simulink model "double_pendulum_model"  (R2022a)
settings: Solver=VariableStepAuto  StartTime=0.0  StopTime=10.0  MaxStep=1/60  RelTol=1e-3  AbsTol=1e-3  EnableMultiTasking=on
undefined symbols (not defined in the file): X, Y, Z
libraries: sm_lib x15, nesl_utility x9, slpidlib x2
settings Model: Creator=tripa  LastModifiedBy=tripa
settings SolverCC: AutoScaleAbsTol=off  AlgebraicLoopSolver=TrustRegion  MaxZcPerStep=1
settings DataIOCC: LimitDataPoints=on  MaxDataPoints=10000
settings OptimizationCC: LifeSpan=inf
settings DebuggingCC: UnconnectedInputMsg=warning  UnconnectedOutputMsg=warning  UnconnectedLineMsg=warning  AllowSymbolicDim=off  SFUnexpectedBacktrackingDiag=warning  SFNoUnconditionalDefaultTransitionDiag=warning  SFExecutionAtInitializationDiag=none  SFMachineParentedDataDiag=warning  ArithmeticOperatorsInVariantConditions=warning
settings SFSimCC: SimUseLocalCustomCode=off  CustomCodeUndefinedFunction=UseInterfaceOnly
settings RTWCC: RTWUseLocalCustomCode=off  DLArmComputeVersion=19.05
settings CodeAppCC: StateflowObjectComments=on
settings GRTTargetCC: TargetLangStandard=C89/C90 (ANSI)
settings ConfigComp: CovMetricSettings=dw  CovSaveCumulativeToWorkspaceVar=on  CovSaveSingleToWorkspaceVar=on  CovExternalEMLEnable=off  CovSFcnEnable=off
settings SimscapeCC: SimscapeLogType=all  SimscapeLogSimulationStatistics=on  SimscapeLogDataHistory=10000

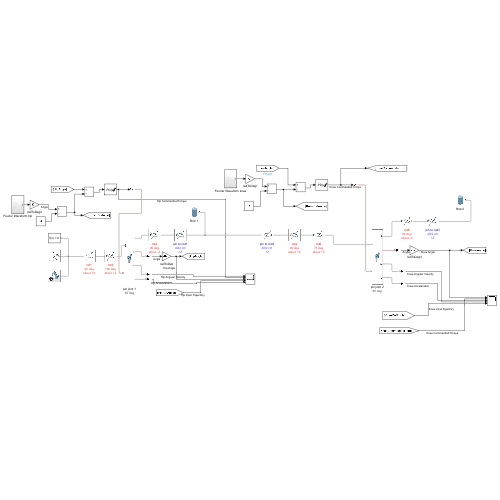
[thumbnail: Simulink's stored preview of the top-level diagram]
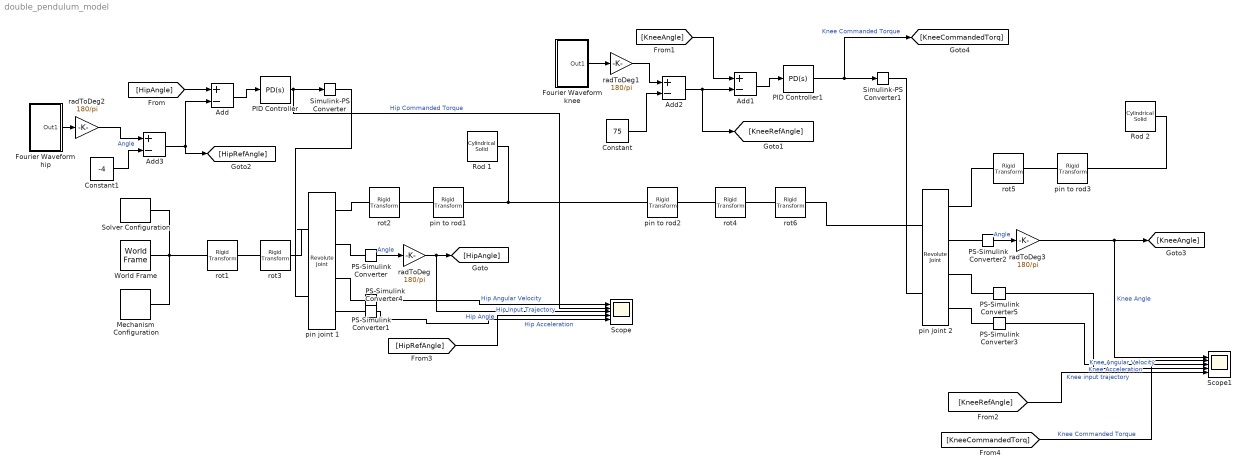
== system double_pendulum_model ==
  Add{,1..3} (4 alike) : Sum  Inputs=+-
  Constant : Constant  Value=75  SampleTime=-1
  Constant1 : Constant  Value=-4  SampleTime=-1
  Fourier Waveform hip : Subsystem
  Fourier Waveform knee : Subsystem
  Mechanism Configuration : sm_lib/Utilities/Mechanism Configuration  UniformGravity=Constant  GravityVector=[0 0 -9.81]  GravityUnits=m/s^2  LinearizationDelta=0.001  JointModeTransitionNonlinearIterations=2
  PID Controller : slpidlib/PID Controller  Controller=PD  Form=Parallel  TimeDomain=Continuous-time  UseExternalTs=off  SampleTime=-1  IntegratorMethod=Forward Euler  FilterMethod=Forward Euler  ControllerParametersSource=internal  P=-23.3308490537665  I=-3.87247530193336  UseKiTs=off  D=-1.5  N=1747.15655402676  UseFilter=on  TunerSelectOption=Transfer Function Based (PID Tuner App)  InitialConditionSource=internal  InitialConditionForIntegrator=0  InitialConditionForFilter=0  DifferentiatorICPrevScaledInput=0  ExternalReset=none  TrackingMode=off  Kt=1  LimitOutput=on  SatLimitsSource=internal  UpperSaturationLimit=20  LowerSaturationLimit=-20  LinearizeAsGain=on  AntiWindupMode=none  Kb=1  POutMin=[]  POutMax=[]  IOutMin=[]  IOutMax=[]  DOutMin=[]  DOutMax=[]  NOutMin=[]  NOutMax=[]  SumOutMin=[]  SumOutMax=[]  SaturationOutMin=[]  SaturationOutMax=[]  PParamMin=[]  PParamMax=[]  IParamMin=[]  IParamMax=[]  DParamMin=[]  DParamMax=[]  NParamMin=[]  NParamMax=[]  KbParamMin=[]  KbParamMax=[]  KtParamMin=[]  KtParamMax=[]  KbOutMin=[]  KbOutMax=[]  KtOutMin=[]  KtOutMax=[]  IntegratorOutMin=[]  IntegratorOutMax=[]  FilterOutMin=[]  FilterOutMax=[]  SumI1OutMin=[]  SumI1OutMax=[]  SumI2OutMin=[]  SumI2OutMax=[]  SumI3OutMin=[]  SumI3OutMax=[]  SumI4OutMin=[]  SumI4OutMax=[]  SumDOutMin=[]  SumDOutMax=[]  DifferentiatorOutMin=[]  DifferentiatorOutMax=[]  FilterDiffOutCoefMin=[]  FilterDiffOutCoefMax=[]  ReciprocalOutMin=[]  ReciprocalOutMax=[]  SumDenOutMin=[]  SumDenOutMax=[]  SumNumOutMin=[]  SumNumOutMax=[]  DivideOutMin=[]  DivideOutMax=[]  UdiffTsProdOutMin=[]  UdiffTsProdOutMax=[]  NTsProdOutMin=[]  NTsProdOutMax=[]  UintegralTsProdOutMin=[]  UintegralTsProdOutMax=[]  UngainTsProdOutMin=[]  UngainTsProdOutMax=[]  IntegratorContinuousStateAttributes=''  IntegratorStateMustResolveToSignalObject=off  IntegratorRTWStateStorageClass=Auto  FilterContinuousStateAttributes=''  FilterStateMustResolveToSignalObject=off  FilterRTWStateStorageClass=Auto  ParallelPVariant=InternalParameters  IdealPVariant=Disabled  IVariant=Disabled  DVariant=InternalParameters  IntegratorVariant=Disabled  SatVariant=Enabled  AWVariant=Disabled  PCopyVariant=Disabled  TRVariant=Disabled  FdbkBlocksVariant=Forward  IdealPFdbkVariant=Disabled  SatFdbkVariant=Disabled  DerivativeFilterVariant=ContFilter  NVariant=InternalParameters  NCopyVariant=Disabled  FilterICVariant=InternalICsFilter  IntegratorICVariant=Disabled  ExternalResetVariant=Disabled  TRSumVariant=Passthrough  SumFdbkVariant=Disabled  SumVariant=Sum_PD  TsampFilterVariant=InternalTs  TsampNgainVariant=Passthrough  TsampIntegralVariant=Disabled_SignalSpec  ExternalSaturationOutDataTypeStr=Inherit: Same as second input  aMode=0
  PID Controller1 : slpidlib/PID Controller  Controller=PD  Form=Parallel  TimeDomain=Continuous-time  UseExternalTs=off  SampleTime=-1  IntegratorMethod=Forward Euler  FilterMethod=Forward Euler  ControllerParametersSource=internal  P=-24.553266008043  I=-3.87247530193336  UseKiTs=off  D=-0.217820826801744  N=2156.83917251684  UseFilter=on  TunerSelectOption=Transfer Function Based (PID Tuner App)  InitialConditionSource=internal  InitialConditionForIntegrator=0  InitialConditionForFilter=0  DifferentiatorICPrevScaledInput=0  ExternalReset=none  TrackingMode=off  Kt=1  LimitOutput=on  SatLimitsSource=internal  UpperSaturationLimit=15  LowerSaturationLimit=-15  LinearizeAsGain=on  AntiWindupMode=none  Kb=1  POutMin=[]  POutMax=[]  IOutMin=[]  IOutMax=[]  DOutMin=[]  DOutMax=[]  NOutMin=[]  NOutMax=[]  SumOutMin=[]  SumOutMax=[]  SaturationOutMin=[]  SaturationOutMax=[]  PParamMin=[]  PParamMax=[]  IParamMin=[]  IParamMax=[]  DParamMin=[]  DParamMax=[]  NParamMin=[]  NParamMax=[]  KbParamMin=[]  KbParamMax=[]  KtParamMin=[]  KtParamMax=[]  KbOutMin=[]  KbOutMax=[]  KtOutMin=[]  KtOutMax=[]  IntegratorOutMin=[]  IntegratorOutMax=[]  FilterOutMin=[]  FilterOutMax=[]  SumI1OutMin=[]  SumI1OutMax=[]  SumI2OutMin=[]  SumI2OutMax=[]  SumI3OutMin=[]  SumI3OutMax=[]  SumI4OutMin=[]  SumI4OutMax=[]  SumDOutMin=[]  SumDOutMax=[]  DifferentiatorOutMin=[]  DifferentiatorOutMax=[]  FilterDiffOutCoefMin=[]  FilterDiffOutCoefMax=[]  ReciprocalOutMin=[]  ReciprocalOutMax=[]  SumDenOutMin=[]  SumDenOutMax=[]  SumNumOutMin=[]  SumNumOutMax=[]  DivideOutMin=[]  DivideOutMax=[]  UdiffTsProdOutMin=[]  UdiffTsProdOutMax=[]  NTsProdOutMin=[]  NTsProdOutMax=[]  UintegralTsProdOutMin=[]  UintegralTsProdOutMax=[]  UngainTsProdOutMin=[]  UngainTsProdOutMax=[]  IntegratorContinuousStateAttributes=''  IntegratorStateMustResolveToSignalObject=off  IntegratorRTWStateStorageClass=Auto  FilterContinuousStateAttributes=''  FilterStateMustResolveToSignalObject=off  FilterRTWStateStorageClass=Auto  ParallelPVariant=InternalParameters  IdealPVariant=Disabled  IVariant=Disabled  DVariant=InternalParameters  IntegratorVariant=Disabled  SatVariant=Enabled  AWVariant=Disabled  PCopyVariant=Disabled  TRVariant=Disabled  FdbkBlocksVariant=Forward  IdealPFdbkVariant=Disabled  SatFdbkVariant=Disabled  DerivativeFilterVariant=ContFilter  NVariant=InternalParameters  NCopyVariant=Disabled  FilterICVariant=InternalICsFilter  IntegratorICVariant=Disabled  ExternalResetVariant=Disabled  TRSumVariant=Passthrough  SumFdbkVariant=Disabled  SumVariant=Sum_PD  TsampFilterVariant=InternalTs  TsampNgainVariant=Passthrough  TsampIntegralVariant=Disabled_SignalSpec  ExternalSaturationOutDataTypeStr=Inherit: Same as second input  aMode=0
  PS-Simulink Converter{,1..5} (6 alike) : nesl_utility/PS-Simulink Converter  PhysicalDomain=network_engine_domain  SubClassName=ps_output  LeftPortType=input  RightPortType=output  PseudoPeriodic=off  Frequencies=[]  VectorFormat=inherit  Unit=inherit  AffineConversion=off
      settings: SourceProductBaseCode=SS,PW,VE
  Rod 1 : sm_lib/Body Elements/Cylindrical Solid  GraphicAmbientColor=[0.15 0.15 0.15 1.0]  BasedOnType=Density  CenterOfMass=[0 0 0]  CenterOfMassUnits=m  GraphicDiffuseColor=[0.5 0.5 0.5]  CylinderLength=40  CylinderLengthUnits=cm  CylinderRadius=3  CylinderRadiusUnits=cm  Density=2700  DensityUnits=kg/m^3  DoExposeReferenceFrame=on  GraphicEmissiveColor=[0.0 0.0 0.0 1.0]  ExportEntireGeometry=off  SerializedFrames=<Frames/>  MarkerShape=Sphere  MarkerSize=10  GraphicType=FromGeometry  InertiaType=CalculateFromGeometry  Mass=1  MassUnits=kg  MomentsOfInertia=[1 1 1]  MomentsOfInertiaUnits=kg*m^2  GraphicOpacity=1.0  ProductsOfInertia=[0 0 0]  ProductsOfInertiaUnits=kg*m^2  GraphicShininess=75  GraphicSpecularColor=[0.5 0.5 0.5 1.0]  GraphicVisPropType=SimpleVisualProperties
  Rod 2 : sm_lib/Body Elements/Cylindrical Solid  GraphicAmbientColor=[0.15 0.15 0.15 1.0]  BasedOnType=Density  CenterOfMass=[0 0 0]  CenterOfMassUnits=m  GraphicDiffuseColor=[0.5 0.5 0.5]  CylinderLength=40  CylinderLengthUnits=cm  CylinderRadius=3  CylinderRadiusUnits=cm  Density=2700  DensityUnits=kg/m^3  DoExposeReferenceFrame=on  GraphicEmissiveColor=[0.0 0.0 0.0 1.0]  ExportEntireGeometry=off  SerializedFrames=<Frames/>  MarkerShape=Sphere  MarkerSize=10  GraphicType=FromGeometry  InertiaType=CalculateFromGeometry  Mass=1  MassUnits=kg  MomentsOfInertia=[1 1 1]  MomentsOfInertiaUnits=kg*m^2  GraphicOpacity=1.0  ProductsOfInertia=[0 0 0]  ProductsOfInertiaUnits=kg*m^2  GraphicShininess=75  GraphicSpecularColor=[0.5 0.5 0.5 1.0]  GraphicVisPropType=SimpleVisualProperties
  Scope : Scope  NumInputPorts=5
  Scope1 : Scope  NumInputPorts=5
  Simulink-PS Converter : nesl_utility/Simulink-PS Converter  PhysicalDomain=network_engine_domain  SubClassName=ps_input  LeftPortType=input  RightPortType=output  PseudoPeriodic=off  Frequencies=[]  NoiseDistribution=none  NoiseParameters=[]  Unit=1  AffineConversion=off  FilteringAndDerivatives=provide  SimscapeFilterOrder=1  InputFilterTimeConstant=0.001  UdotUserProvided=0
      settings: SourceProductBaseCode=SS,PW,VE
  Simulink-PS Converter1 : nesl_utility/Simulink-PS Converter  PhysicalDomain=network_engine_domain  SubClassName=ps_input  LeftPortType=input  RightPortType=output  PseudoPeriodic=off  Frequencies=[]  NoiseDistribution=none  NoiseParameters=[]  Unit=1  AffineConversion=off  FilteringAndDerivatives=provide  SimscapeFilterOrder=1  InputFilterTimeConstant=0.001  UdotUserProvided=0
      settings: SourceProductBaseCode=SS,PW,VE
  Solver Configuration : nesl_utility/Solver Configuration  PhysicalDomain=network_engine_domain  SubClassName=solver  LeftPortType=input  RightPortType=generic  Tones=[]  Harmonics=[]  SimulateNoise=off  Profile=off  UseLocalSampling=off  EnableSwitchedLinearOptims=on  FrequencyDomain=off  UseCCode=off  RelTol=0.001  AbsTol=1e-06  MinStep=1e-09  ToWorkspace=off  RevertToSquareIcSolve=off  NumHomotopyIterations=100  PhasorMode=off  PhasorModeNumHarmonics=1  IndexReductionMethod=DerivativeReplacement  DoDC=off  ResidualTolerance=1e-09  UseLocalSolver=off  LocalSolverChoice=NE_BACKWARD_EULER_ADVANCER  LocalSolverSampleTime=0.001  DoFixedCost=off  MaxNonlinIter=3  MaxModeIter=2  ComputeImpulses=off  ImpulseIterations=2  LinearAlgebra=Sparse  LinearAlgebraNumThread=0  EquationFormulation=NE_TIME_EF  DelaysMemoryBudget=1024  AutomaticFiltering=on  FilteringTimeConstant=0.001  PartitionStorageMethod=AS_NEEDED  PartitionMemoryBudget=1024  PartitionMethod=FAST
      settings: SourceProductBaseCode=SS,PW,VE
  World Frame : sm_lib/Frames and Transforms/World Frame
  pin joint 1 : sm_lib/Joints/Revolute Joint  JointMode=Normal  SenseConstraintForce=off  SenseConstraintForceX=off  SenseConstraintForceY=off  SenseConstraintForceZ=off  SenseConstraintTorque=off  SenseConstraintTorqueX=off  SenseConstraintTorqueY=off  SenseConstraintTorqueZ=off  SenseTotalForce=off  SenseTotalForceX=off  SenseTotalForceY=off  SenseTotalForceZ=off  SenseTotalTorque=off  SenseTotalTorqueX=off  SenseTotalTorqueY=off  SenseTotalTorqueZ=off  CompositeWrenchDir=FollowerOnBase  CompositeWrenchFrame=BaseFrame  EquilibriumPosition=0  EquilibriumPositionUnits=deg  SpringStiffness=0  SpringStiffnessUnits=N*m/deg  DampingCoefficient=0  DampingCoefficientUnits=N*m/(deg/s)  TorqueActuationMode=InputTorque  MotionActuationMode=ComputedMotion  SensePosition=on  SenseVelocity=on  SenseAcceleration=on  SenseTorqueForce=off  SenseLowerLimitTorqueForce=off  SenseUpperLimitTorqueForce=off  LowerLimitSpecify=off  LowerLimitBound=-90  LowerLimitBoundUnits=deg  LowerLimitStiffness=1e4  LowerLimitStiffnessUnits=N*m/deg  LowerLimitDamping=10  LowerLimitDampingUnits=N*m/(deg/s)  LowerLimitTransitionRegionWidth=0.1  LowerLimitTransitionRegionWidthUnits=deg  UpperLimitSpecify=off  UpperLimitBound=90  UpperLimitBoundUnits=deg  UpperLimitStiffness=1e4  UpperLimitStiffnessUnits=N*m/deg  UpperLimitDamping=10  UpperLimitDampingUnits=N*m/(deg/s)  UpperLimitTransitionRegionWidth=0.1  UpperLimitTransitionRegionWidthUnits=deg  PositionTargetSpecify=off  PositionTargetPriority=High  PositionTargetValue=90  PositionTargetValueUnits=deg  VelocityTargetSpecify=off  VelocityTargetPriority=High  VelocityTargetValue=0  VelocityTargetValueUnits=deg/s
      settings: AttributesFormatString=%<PositionTargetValue> %<PositionTargetValueUnits>
  pin joint 2 : sm_lib/Joints/Revolute Joint  JointMode=Normal  SenseConstraintForce=off  SenseConstraintForceX=off  SenseConstraintForceY=off  SenseConstraintForceZ=off  SenseConstraintTorque=off  SenseConstraintTorqueX=off  SenseConstraintTorqueY=off  SenseConstraintTorqueZ=off  SenseTotalForce=off  SenseTotalForceX=off  SenseTotalForceY=off  SenseTotalForceZ=off  SenseTotalTorque=off  SenseTotalTorqueX=off  SenseTotalTorqueY=off  SenseTotalTorqueZ=off  CompositeWrenchDir=FollowerOnBase  CompositeWrenchFrame=BaseFrame  EquilibriumPosition=0  EquilibriumPositionUnits=deg  SpringStiffness=0  SpringStiffnessUnits=N*m/deg  DampingCoefficient=0  DampingCoefficientUnits=N*m/(deg/s)  TorqueActuationMode=InputTorque  MotionActuationMode=ComputedMotion  SensePosition=on  SenseVelocity=on  SenseAcceleration=on  SenseTorqueForce=off  SenseLowerLimitTorqueForce=off  SenseUpperLimitTorqueForce=off  LowerLimitSpecify=off  LowerLimitBound=-90  LowerLimitBoundUnits=deg  LowerLimitStiffness=1e4  LowerLimitStiffnessUnits=N*m/deg  LowerLimitDamping=10  LowerLimitDampingUnits=N*m/(deg/s)  LowerLimitTransitionRegionWidth=0.1  LowerLimitTransitionRegionWidthUnits=deg  UpperLimitSpecify=off  UpperLimitBound=90  UpperLimitBoundUnits=deg  UpperLimitStiffness=1e4  UpperLimitStiffnessUnits=N*m/deg  UpperLimitDamping=10  UpperLimitDampingUnits=N*m/(deg/s)  UpperLimitTransitionRegionWidth=0.1  UpperLimitTransitionRegionWidthUnits=deg  PositionTargetSpecify=off  PositionTargetPriority=High  PositionTargetValue=90  PositionTargetValueUnits=deg  VelocityTargetSpecify=off  VelocityTargetPriority=High  VelocityTargetValue=0  VelocityTargetValueUnits=deg/s
      settings: AttributesFormatString=%<PositionTargetValue> %<PositionTargetValueUnits>
  pin to rod1 : sm_lib/Frames and Transforms/Rigid Transform  TranslationMethod=StandardAxis  TranslationStandardOffset=40/2  TranslationLengthUnit=cm  TranslationStandardAxis=+Z  TranslationCartesianOffset=[0 0 0]  TranslationROffset=0  TranslationROffsetUnits=m  TranslationZOffset=0  TranslationZOffsetUnits=m  TranslationThetaOffset=0  TranslationThetaOffsetUnits=deg  RotationMethod=None  RotationAngleUnits=deg  RotationStandardAxis=+X  RotationAngle=90  RotationArbitraryAxis=[0 0 1]  FollAlignAxisA=+X  BaseAlignAxisA=+Y  FollAlignAxisB=+Y  BaseAlignAxisB=+Z  RotationSequenceAxes=FollowerAxes  RotationSequence=XYX  RotationSequenceAngles=[0 0 0]  RotationSequenceAnglesUnits=deg  RotationMatrix=[1 0 0; 0 1 0; 0 0 1]
      settings: AttributesFormatString=|
      | %<TranslationStandardOffset> %<TranslationLengthUnit>
      | %<TranslationStandardAxis>
  pin to rod2 : sm_lib/Frames and Transforms/Rigid Transform  TranslationMethod=StandardAxis  TranslationStandardOffset=40/2  TranslationLengthUnit=cm  TranslationStandardAxis=+Z  TranslationCartesianOffset=[0 0 0]  TranslationROffset=0  TranslationROffsetUnits=m  TranslationZOffset=0  TranslationZOffsetUnits=m  TranslationThetaOffset=0  TranslationThetaOffsetUnits=deg  RotationMethod=None  RotationAngleUnits=deg  RotationStandardAxis=+X  RotationAngle=90  RotationArbitraryAxis=[0 0 1]  FollAlignAxisA=+X  BaseAlignAxisA=+Y  FollAlignAxisB=+Y  BaseAlignAxisB=+Z  RotationSequenceAxes=FollowerAxes  RotationSequence=XYX  RotationSequenceAngles=[0 0 0]  RotationSequenceAnglesUnits=deg  RotationMatrix=[1 0 0; 0 1 0; 0 0 1]
      settings: AttributesFormatString=|
      | %<TranslationStandardOffset> %<TranslationLengthUnit>
      | %<TranslationStandardAxis>
  pin to rod3 : sm_lib/Frames and Transforms/Rigid Transform  TranslationMethod=StandardAxis  TranslationStandardOffset=40/2  TranslationLengthUnit=cm  TranslationStandardAxis=+Z  TranslationCartesianOffset=[0 0 0]  TranslationROffset=0  TranslationROffsetUnits=m  TranslationZOffset=0  TranslationZOffsetUnits=m  TranslationThetaOffset=0  TranslationThetaOffsetUnits=deg  RotationMethod=None  RotationAngleUnits=deg  RotationStandardAxis=+X  RotationAngle=90  RotationArbitraryAxis=[0 0 1]  FollAlignAxisA=+X  BaseAlignAxisA=+Y  FollAlignAxisB=+Y  BaseAlignAxisB=+Z  RotationSequenceAxes=FollowerAxes  RotationSequence=XYX  RotationSequenceAngles=[0 0 0]  RotationSequenceAnglesUnits=deg  RotationMatrix=[1 0 0; 0 1 0; 0 0 1]
      settings: AttributesFormatString=|
      | %<TranslationStandardOffset> %<TranslationLengthUnit>
      | %<TranslationStandardAxis>
  radToDeg{,1..3} (4 alike) : Gain  Gain=180/pi
  rot1 : sm_lib/Frames and Transforms/Rigid Transform  TranslationMethod=None  TranslationStandardOffset=0  TranslationLengthUnit=m  TranslationStandardAxis=+Z  TranslationCartesianOffset=[0 0 0]  TranslationROffset=0  TranslationROffsetUnits=m  TranslationZOffset=0  TranslationZOffsetUnits=m  TranslationThetaOffset=0  TranslationThetaOffsetUnits=deg  RotationMethod=StandardAxis  RotationAngleUnits=deg  RotationStandardAxis=+X  RotationAngle=90  RotationArbitraryAxis=[0 0 1]  FollAlignAxisA=+X  BaseAlignAxisA=+Y  FollAlignAxisB=+Y  BaseAlignAxisB=+Z  RotationSequenceAxes=FollowerAxes  RotationSequence=XYX  RotationSequenceAngles=[0 0 0]  RotationSequenceAnglesUnits=deg  RotationMatrix=[1 0 0; 0 1 0; 0 0 1]
      settings: AttributesFormatString=|
      | %<RotationAngle> %<RotationAngleUnits>
      | about %<RotationStandardAxis>
  rot2 : sm_lib/Frames and Transforms/Rigid Transform  TranslationMethod=None  TranslationStandardOffset=0  TranslationLengthUnit=m  TranslationStandardAxis=+Z  TranslationCartesianOffset=[0 0 0]  TranslationROffset=0  TranslationROffsetUnits=m  TranslationZOffset=0  TranslationZOffsetUnits=m  TranslationThetaOffset=0  TranslationThetaOffsetUnits=deg  RotationMethod=StandardAxis  RotationAngleUnits=deg  RotationStandardAxis=-X  RotationAngle=90  RotationArbitraryAxis=[0 0 1]  FollAlignAxisA=+X  BaseAlignAxisA=+Y  FollAlignAxisB=+Y  BaseAlignAxisB=+Z  RotationSequenceAxes=FollowerAxes  RotationSequence=XYX  RotationSequenceAngles=[0 0 0]  RotationSequenceAnglesUnits=deg  RotationMatrix=[1 0 0; 0 1 0; 0 0 1]
      settings: AttributesFormatString=|
      | %<RotationAngle> %<RotationAngleUnits>
      | about %<RotationStandardAxis>
  rot3 : sm_lib/Frames and Transforms/Rigid Transform  TranslationMethod=None  TranslationStandardOffset=0  TranslationLengthUnit=m  TranslationStandardAxis=+Z  TranslationCartesianOffset=[0 0 0]  TranslationROffset=0  TranslationROffsetUnits=m  TranslationZOffset=0  TranslationZOffsetUnits=m  TranslationThetaOffset=0  TranslationThetaOffsetUnits=deg  RotationMethod=StandardAxis  RotationAngleUnits=deg  RotationStandardAxis=+Z  RotationAngle=180  RotationArbitraryAxis=[0 0 1]  FollAlignAxisA=+X  BaseAlignAxisA=+Y  FollAlignAxisB=+Y  BaseAlignAxisB=+Z  RotationSequenceAxes=FollowerAxes  RotationSequence=XYX  RotationSequenceAngles=[0 0 0]  RotationSequenceAnglesUnits=deg  RotationMatrix=[1 0 0; 0 1 0; 0 0 1]
      settings: AttributesFormatString=|
      | %<RotationAngle> %<RotationAngleUnits>
      | about %<RotationStandardAxis>
  rot4 : sm_lib/Frames and Transforms/Rigid Transform  TranslationMethod=None  TranslationStandardOffset=0  TranslationLengthUnit=m  TranslationStandardAxis=+Z  TranslationCartesianOffset=[0 0 0]  TranslationROffset=0  TranslationROffsetUnits=m  TranslationZOffset=0  TranslationZOffsetUnits=m  TranslationThetaOffset=0  TranslationThetaOffsetUnits=deg  RotationMethod=StandardAxis  RotationAngleUnits=deg  RotationStandardAxis=+X  RotationAngle=90  RotationArbitraryAxis=[0 0 1]  FollAlignAxisA=+X  BaseAlignAxisA=+Y  FollAlignAxisB=+Y  BaseAlignAxisB=+Z  RotationSequenceAxes=FollowerAxes  RotationSequence=XYX  RotationSequenceAngles=[0 0 0]  RotationSequenceAnglesUnits=deg  RotationMatrix=[1 0 0; 0 1 0; 0 0 1]
      settings: AttributesFormatString=|
      | %<RotationAngle> %<RotationAngleUnits>
      | about %<RotationStandardAxis>
  rot5 : sm_lib/Frames and Transforms/Rigid Transform  TranslationMethod=None  TranslationStandardOffset=0  TranslationLengthUnit=m  TranslationStandardAxis=+Z  TranslationCartesianOffset=[0 0 0]  TranslationROffset=0  TranslationROffsetUnits=m  TranslationZOffset=0  TranslationZOffsetUnits=m  TranslationThetaOffset=0  TranslationThetaOffsetUnits=deg  RotationMethod=StandardAxis  RotationAngleUnits=deg  RotationStandardAxis=-X  RotationAngle=90  RotationArbitraryAxis=[0 0 1]  FollAlignAxisA=+X  BaseAlignAxisA=+Y  FollAlignAxisB=+Y  BaseAlignAxisB=+Z  RotationSequenceAxes=FollowerAxes  RotationSequence=XYX  RotationSequenceAngles=[0 0 0]  RotationSequenceAnglesUnits=deg  RotationMatrix=[1 0 0; 0 1 0; 0 0 1]
      settings: AttributesFormatString=|
      | %<RotationAngle> %<RotationAngleUnits>
      | about %<RotationStandardAxis>
  rot6 : sm_lib/Frames and Transforms/Rigid Transform  TranslationMethod=None  TranslationStandardOffset=0  TranslationLengthUnit=m  TranslationStandardAxis=+Z  TranslationCartesianOffset=[0 0 0]  TranslationROffset=0  TranslationROffsetUnits=m  TranslationZOffset=0  TranslationZOffsetUnits=m  TranslationThetaOffset=0  TranslationThetaOffsetUnits=deg  RotationMethod=StandardAxis  RotationAngleUnits=deg  RotationStandardAxis=+Z  RotationAngle=75  RotationArbitraryAxis=[0 0 1]  FollAlignAxisA=+X  BaseAlignAxisA=+Y  FollAlignAxisB=+Y  BaseAlignAxisB=+Z  RotationSequenceAxes=FollowerAxes  RotationSequence=XYX  RotationSequenceAngles=[0 0 0]  RotationSequenceAnglesUnits=deg  RotationMatrix=[1 0 0; 0 1 0; 0 0 1]
      settings: AttributesFormatString=|
      | %<RotationAngle> %<RotationAngleUnits>
      | about %<RotationStandardAxis>
  wires:
  PS-Simulink Converter/1 -> radToDeg/1  "Angle"
  PS-Simulink Converter1/1 -> Scope/1  "Hip Angular Velocity"
  radToDeg/1 -> Scope/3, [HipAngle]  "Hip Angle"
  PID Controller/1 -> Simulink-PS Converter/1, Scope/2  "Hip Commanded Torque"
  [HipAngle] -> Add/1
  Add/1 -> PID Controller/1
  PS-Simulink Converter4/1 -> Scope/5  "Hip Acceleration"
  [HipRefAngle] -> Scope/4  "Hip Input Trajectory"
  Fourier Waveform hip/1(Out1) -> radToDeg2/1
  Fourier Waveform knee/1(Out1) -> radToDeg1/1
  Add1/1 -> PID Controller1/1
  [KneeAngle] -> Add1/1
  PID Controller1/1 -> [KneeCommandedTorq], Simulink-PS Converter1/1  "Knee Commanded Torque"
  [KneeRefAngle] -> Scope1/5  "Knee input trajectory"
  PS-Simulink Converter2/1 -> radToDeg3/1  "Angle"
  radToDeg3/1 -> Scope1/1, [KneeAngle]  "Knee Angle"
  PS-Simulink Converter5/1 -> Scope1/4  "Knee Angular Velocity"
  PS-Simulink Converter3/1 -> Scope1/3  "Knee Acceleration"
  [KneeCommandedTorq] -> Scope1/2  "Knee Commanded Torque"
  radToDeg1/1 -> Add2/1
  Add2/1 -> [KneeRefAngle], Add1/2
  Constant/1 -> Add2/2
  radToDeg2/1 -> Add3/1  "Angle"
  Constant1/1 -> Add3/2
  Add3/1 -> [HipRefAngle], Add/2
  connections:
  World Frame/RConn1 -- rot1/LConn1 -- Solver Configuration/RConn1 -- Mechanism Configuration/RConn1
  pin joint 1/LConn1 -- rot3/RConn1
  PS-Simulink Converter/LConn1 -- pin joint 1/RConn2
  PS-Simulink Converter1/LConn1 -- pin joint 1/RConn3
  pin joint 1/RConn1 -- rot2/LConn1
  rot2/RConn1 -- pin to rod1/LConn1
  pin to rod1/RConn1 -- pin to rod2/LConn1 -- Rod 1/RConn1
  rot3/LConn1 -- rot1/RConn1
  Simulink-PS Converter/RConn1 -- pin joint 1/LConn2
  PS-Simulink Converter4/LConn1 -- pin joint 1/RConn4
  pin to rod2/RConn1 -- rot4/LConn1
  rot4/RConn1 -- rot6/LConn1
  Simulink-PS Converter1/RConn1 -- pin joint 2/LConn2
  rot5/LConn1 -- pin joint 2/RConn1
  rot5/RConn1 -- pin to rod3/LConn1
  PS-Simulink Converter2/LConn1 -- pin joint 2/RConn2
  pin to rod3/RConn1 -- Rod 2/RConn1
  pin joint 2/RConn4 -- PS-Simulink Converter3/LConn1
  pin joint 2/RConn3 -- PS-Simulink Converter5/LConn1
  rot6/RConn1 -- pin joint 2/LConn1

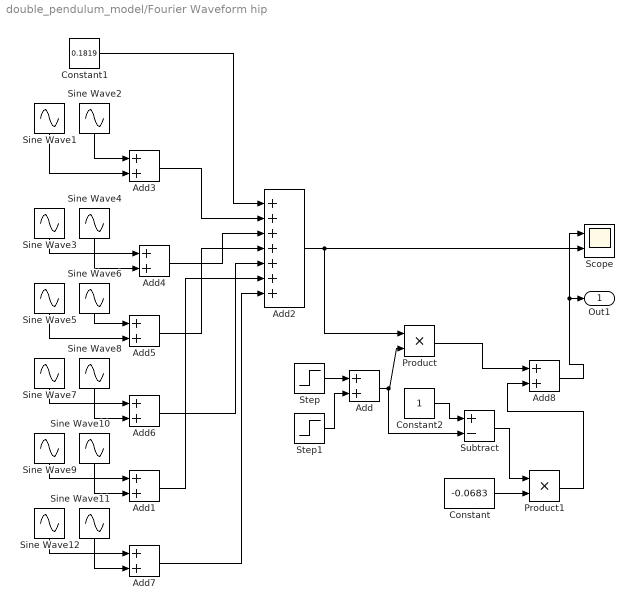
== system double_pendulum_model/Fourier Waveform hip ==
  Add{,1,3..8} (8 alike) : Sum
  Add2 : Sum  Inputs=+++++++
  Constant : Constant  Value=-0.0683  SampleTime=-1
  Constant1 : Constant  Value=0.1819  SampleTime=-1
  Constant2 : Constant  SampleTime=-1
  Product : Product
  Product1 : Product
  Scope : Scope  NumInputPorts=2
  Sine Wave1 : Sin  Amplitude=-0.2755  Frequency=4.424  Phase=pi/2  SampleTime=0
  Sine Wave10 : Sin  Amplitude=0.002542  Frequency=4.424*5  SampleTime=0
  Sine Wave11 : Sin  Amplitude=0.005374  Frequency=4.424*6  SampleTime=0
  Sine Wave12 : Sin  Amplitude=0.001063  Frequency=4.424*6  Phase=pi/2  SampleTime=0
  Sine Wave2 : Sin  Amplitude=0.03057  Frequency=4.424  SampleTime=0
  Sine Wave3 : Sin  Amplitude=-0.02595  Frequency=4.424*2  Phase=pi/2  SampleTime=0
  Sine Wave4 : Sin  Amplitude=-0.04813  Frequency=4.424*2  SampleTime=0
  Sine Wave5 : Sin  Amplitude=0.02598  Frequency=4.424*3  Phase=pi/2  SampleTime=0
  Sine Wave6 : Sin  Amplitude=-0.01268  Frequency=4.424*3  SampleTime=0
  Sine Wave7 : Sin  Amplitude=0.01088  Frequency=4.424*4  Phase=pi/2  SampleTime=0
  Sine Wave8 : Sin  Amplitude=0.002473  Frequency=4.424*4  SampleTime=0
  Sine Wave9 : Sin  Amplitude=0.01099  Frequency=4.424*5  Phase=pi/2  SampleTime=0
  Step : Step  Time=0  SampleTime=0
  Step1 : Step  Time=1.24  After=-1  SampleTime=0
  Subtract : Sum  Inputs=+-
  Out1 : Outport
  wires:
  Add6/1 -> Add2/5
  Constant1/1 -> Add2/1
  Sine Wave2/1 -> Add3/1
  Add3/1 -> Add2/2
  Sine Wave3/1 -> Add4/1
  Sine Wave8/1 -> Add6/2
  Sine Wave6/1 -> Add5/1
  Sine Wave1/1 -> Add3/2
  Sine Wave5/1 -> Add5/2
  Sine Wave4/1 -> Add4/2
  Sine Wave7/1 -> Add6/1
  Add4/1 -> Add2/3
  Add5/1 -> Add2/4
  Add2/1 -> Scope/2, Product/1
  Add1/1 -> Add2/6
  Sine Wave9/1 -> Add1/1
  Sine Wave10/1 -> Add1/2
  Sine Wave11/1 -> Add7/2
  Sine Wave12/1 -> Add7/1
  Add7/1 -> Add2/7
  Add8/1 -> Scope/1, Out1/1
  Step1/1 -> Add/2
  Step/1 -> Add/1
  Add/1 -> Subtract/2, Product/2
  Constant/1 -> Product1/2
  Constant2/1 -> Subtract/1
  Subtract/1 -> Product1/1
  Product1/1 -> Add8/2
  Product/1 -> Add8/1

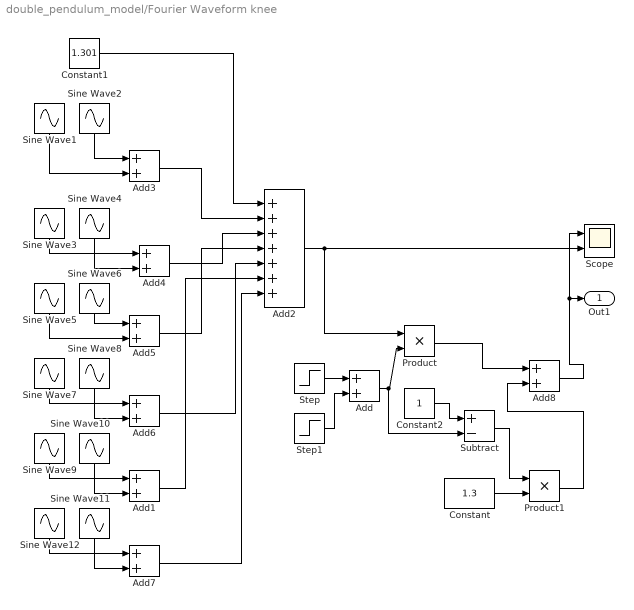
== system double_pendulum_model/Fourier Waveform knee ==
  Add{,1,3..8} (8 alike) : Sum
  Add2 : Sum  Inputs=+++++++
  Constant : Constant  Value=1.3  SampleTime=-1
  Constant1 : Constant  Value=1.301  SampleTime=-1
  Constant2 : Constant  SampleTime=-1
  Product : Product
  Product1 : Product
  Scope : Scope  NumInputPorts=2
  Sine Wave1 : Sin  Amplitude=-0.2874  Frequency=4.528  Phase=pi/2  SampleTime=0
  Sine Wave10 : Sin  Amplitude=-0.0008434  Frequency=4.528*5  SampleTime=0
  Sine Wave11 : Sin  Amplitude=-0.005466  Frequency=4.528*6  SampleTime=0
  Sine Wave12 : Sin  Amplitude=0.005971  Frequency=4.528*6  Phase=pi/2  SampleTime=0
  Sine Wave2 : Sin  Amplitude=-0.3596  Frequency=4.528  SampleTime=0
  Sine Wave3 : Sin  Amplitude=0.2369  Frequency=4.528*2  Phase=pi/2  SampleTime=0
  Sine Wave4 : Sin  Amplitude=-0.01515  Frequency=4.528*2  SampleTime=0
  Sine Wave5 : Sin  Amplitude=-0.04392  Frequency=4.528*3  Phase=pi/2  SampleTime=0
  Sine Wave6 : Sin  Amplitude=0.04249  Frequency=4.528*3  SampleTime=0
  Sine Wave7 : Sin  Amplitude=0.006223  Frequency=4.528*4  Phase=pi/2  SampleTime=0
  Sine Wave8 : Sin  Amplitude=-0.002943  Frequency=4.528*4  SampleTime=0
  Sine Wave9 : Sin  Amplitude=-0.01249  Frequency=4.528*5  Phase=pi/2  SampleTime=0
  Step : Step  Time=0  SampleTime=0
  Step1 : Step  Time=1.24  After=-1  SampleTime=0
  Subtract : Sum  Inputs=+-
  Out1 : Outport
  wires:
  Product/1 -> Add8/1
  Product1/1 -> Add8/2
  Subtract/1 -> Product1/1
  Constant2/1 -> Subtract/1
  Constant/1 -> Product1/2
  Add/1 -> Product/2, Subtract/2
  Step/1 -> Add/1
  Step1/1 -> Add/2
  Add8/1 -> Out1/1, Scope/1
  Add7/1 -> Add2/7
  Sine Wave12/1 -> Add7/1
  Sine Wave11/1 -> Add7/2
  Sine Wave10/1 -> Add1/2
  Sine Wave9/1 -> Add1/1
  Add1/1 -> Add2/6
  Add2/1 -> Product/1, Scope/2
  Add5/1 -> Add2/4
  Add4/1 -> Add2/3
  Sine Wave7/1 -> Add6/1
  Sine Wave4/1 -> Add4/2
  Sine Wave5/1 -> Add5/2
  Sine Wave1/1 -> Add3/2
  Sine Wave6/1 -> Add5/1
  Sine Wave8/1 -> Add6/2
  Sine Wave3/1 -> Add4/1
  Add3/1 -> Add2/2
  Sine Wave2/1 -> Add3/1
  Constant1/1 -> Add2/1
  Add6/1 -> Add2/5
